simulink model "project1sim"  (R2022b)
settings: Solver=VariableStepAuto  StartTime=0.0  StopTime=120  MaxStep=0.001  RelTol=1e-3
values from neighbouring files (symbols this model uses):
  cs = 1500    [LS.m]    (also in RLS.m; project1.m)
  ks = 20000    [project1.m]
  kt = 180000    [LS.m]    (also in RLS.m; project1.m)
  m1 = 250    [project1.m]
  m2 = 40    [LS.m]    (also in RLS.m; project1.m)
libraries: simulink x1
settings Model: Creator=Forough  LastModifiedBy=Forough

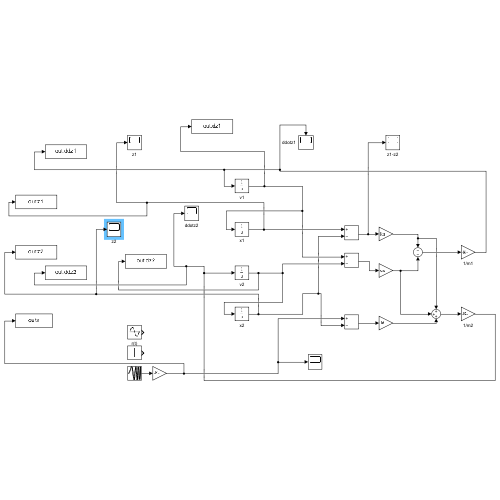
[thumbnail: Simulink's stored preview of the top-level diagram]
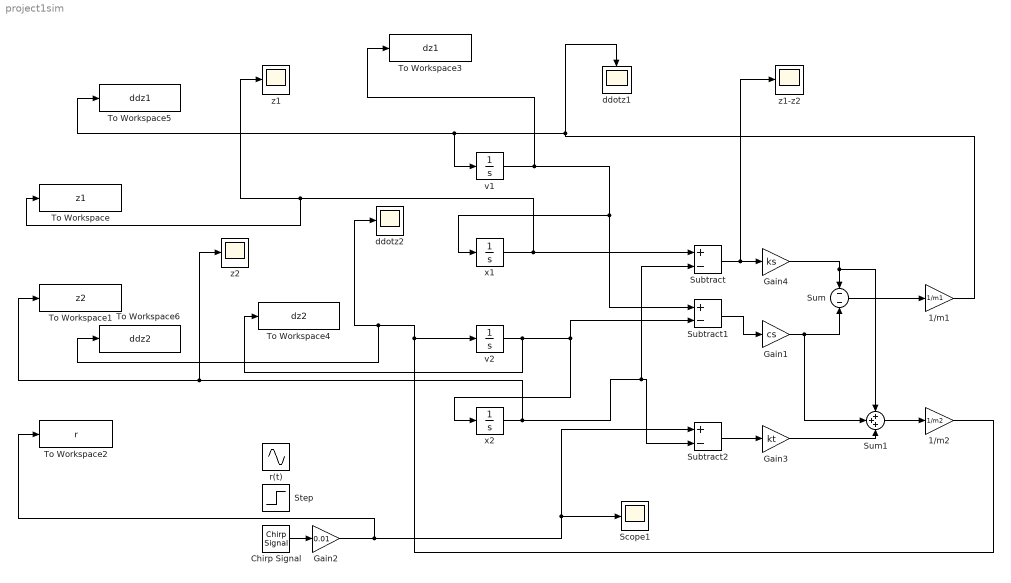
== system project1sim ==
  1/m1 : Gain  Gain=1/m1
  1/m2 : Gain  Gain=1/m2
  Chirp Signal : simulink/Sources/Chirp Signal  f1=1  T=120  f2=10
  Gain1 : Gain  Gain=cs
  Gain2 : Gain  Gain=0.01
  Gain3 : Gain  Gain=kt
  Gain4 : Gain  Gain=ks
  Scope1 : Scope
  Step : Step  After=0.05  SampleTime=0
  Subtract : Sum  Inputs=+-
  Subtract1 : Sum  Inputs=+-
  Subtract2 : Sum  Inputs=+-
  Sum : Sum  Inputs=--
  Sum1 : Sum  Inputs=+++
  To Workspace : ToWorkspace  VariableName=z1  SaveFormat=Timeseries  SampleTime=-1
  To Workspace1 : ToWorkspace  VariableName=z2  SaveFormat=Timeseries  SampleTime=-1
  To Workspace2 : ToWorkspace  VariableName=r  SaveFormat=Timeseries  SampleTime=-1
  To Workspace3 : ToWorkspace  VariableName=dz1  SaveFormat=Timeseries  SampleTime=-1
  To Workspace4 : ToWorkspace  VariableName=dz2  SaveFormat=Timeseries  SampleTime=-1
  To Workspace5 : ToWorkspace  VariableName=ddz1  SaveFormat=Timeseries  SampleTime=-1
  To Workspace6 : ToWorkspace  VariableName=ddz2  SaveFormat=Timeseries  SampleTime=-1
  ddotz1 : Scope
  ddotz2 : Scope
  r(t) : Sin  Amplitude=0.01  Frequency=523.6  SampleTime=0
  v1 : Integrator
  v2 : Integrator
  x1 : Integrator
  x2 : Integrator
  z1 : Scope
  z1-z2 : Scope
  z2 : Scope
  wires:
  Subtract/1 -> Gain4/1, z1-z2/1
  x1/1 -> To Workspace/1, z1/1, Subtract/1
  x2/1 -> To Workspace1/1, z2/1, Subtract/2, Subtract2/2
  v1/1 -> To Workspace3/1, Subtract1/1, x1/1
  v2/1 -> To Workspace4/1, x2/1, Subtract1/2
  Subtract1/1 -> Gain1/1
  Gain4/1 -> Sum1/1, Sum/1
  Gain1/1 -> Sum1/2, Sum/2
  Sum/1 -> 1/m1/1
  Subtract2/1 -> Gain3/1
  Gain3/1 -> Sum1/3
  Sum1/1 -> 1/m2/1
  1/m2/1 -> To Workspace6/1, ddotz2/1, v2/1
  Gain2/1 -> To Workspace2/1, Subtract2/1, Scope1/1
  1/m1/1 -> ddotz1/1, To Workspace5/1, v1/1
  Chirp Signal/1 -> Gain2/1
